simulink model "riseTrigger_twoStateSM"  (R2024b)
settings: Solver=VariableStepAuto  StartTime=0.0  StopTime=10.0  RelTol=1e-3
settings Model: Creator=optimus  LastModifiedBy=optimus

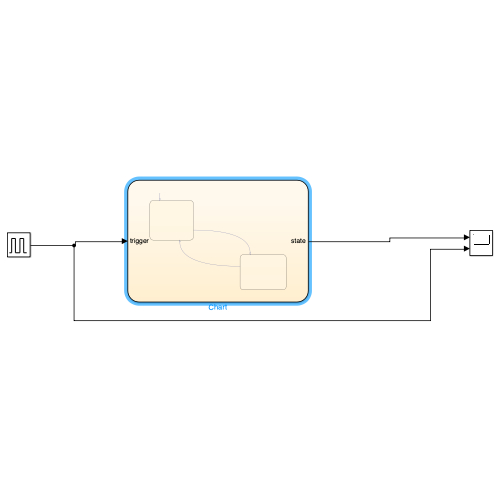
[thumbnail: Simulink's stored preview of the top-level diagram]
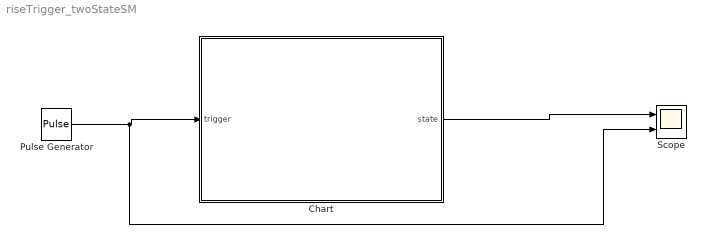
== system riseTrigger_twoStateSM ==
  Chart : Stateflow chart  TreatAsAtomicUnit=on
  Pulse Generator : DiscretePulseGenerator  PulseType=Time based  PulseWidth=50
  Scope : Scope  NumInputPorts=2
  wires:
  Pulse Generator/1 -> Scope/2, Chart/1(trigger)
  Chart/1(state) -> Scope/1

== stateflow chart riseTrigger_twoStateSM/Chart ==
  state A
    entry:
    state=0;
    prev=1;
    during:
    if(trigger==0)
    prev=0;
    end
  state B
    entry:
    state=1;
    prev=1;
    during:
    if(trigger==0)
    prev=0;
    end
  (default) -> A
  A -> B : [trigger==1 && prev==0]
  B -> A : [trigger==1 && prev==0]
  data: state output; trigger input; prev local =0
